simulink model "lab3_nonlinear"  (R2025b)
settings: Solver=VariableStepAuto  StartTime=0.0  StopTime=10.0  RelTol=1e-10  AbsTol=1e-10
values from neighbouring files (symbols this model uses):
  A = double(subs(J1, [x;u], [x_bar;u_bar]))    [lab3.m]
  B = double(subs(J2, [x;u], [x_bar;u_bar]))    [lab3.m]
  K = -K_LQR2    [lab3.m]
  Ulim = 5.875    [lab3.m]
  x0 = [0; 0; 2*pi/24; 0]    [lab3.m]

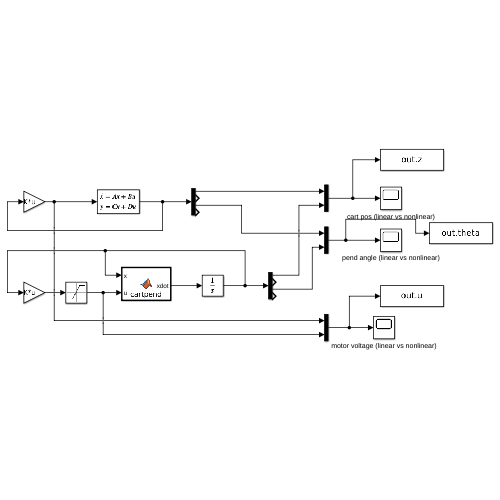
[thumbnail: Simulink's stored preview of the top-level diagram]
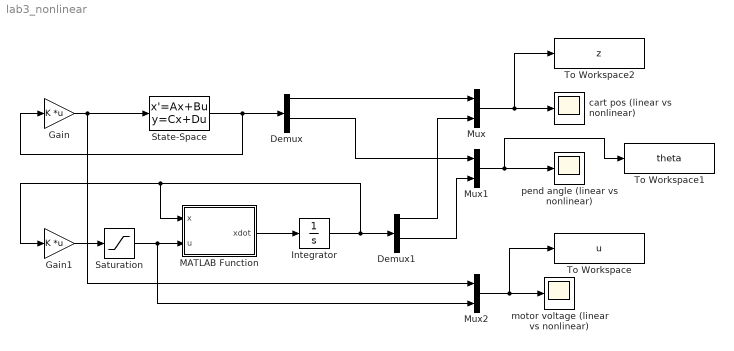
== system lab3_nonlinear ==
  Demux : Demux
  Demux1 : Demux
  Gain : Gain  Gain=K  Multiplication=Matrix(K*u)
  Gain1 : Gain  Gain=K  Multiplication=Matrix(K*u)
  Integrator : Integrator  InitialCondition=x0
  MATLAB Function : MATLAB Function  TreatAsAtomicUnit=on
  Mux : Mux  Inputs=2
  Mux1 : Mux  Inputs=2
  Mux2 : Mux  Inputs=2
  Saturation : Saturate  UpperLimit=Ulim  LowerLimit=-Ulim
  State-Space : StateSpace  A=A  B=B  C=eye(4)  D=zeros(4,1)  InitialCondition=x0
  To Workspace : ToWorkspace  VariableName=u  SaveFormat=Timeseries  SampleTime=-1
  To Workspace1 : ToWorkspace  VariableName=theta  SaveFormat=Timeseries  SampleTime=-1
  To Workspace2 : ToWorkspace  VariableName=z  SaveFormat=Timeseries  SampleTime=-1
  cart pos (linear vs nonlinear) : Scope
      settings: ActiveDisplayYMinimum=-0.12196514215297433  ActiveDisplayYMaximum=-0.023098636726185284
  motor voltage (linear vs nonlinear) : Scope
      settings: DataLoggingVariableName=ScopeData2
  pend angle (linear vs nonlinear) : Scope
      settings: ActiveDisplayYMinimum=-0.089196382902815077  ActiveDisplayYMaximum=0.15535481354428468
  wires:
  Gain/1 -> Mux2/1, State-Space/1
  State-Space/1 -> Gain/1, Demux/1
  Demux/1 -> Mux/1
  Gain1/1 -> Saturation/1
  Saturation/1 -> Mux2/2, MATLAB Function/2(u)
  MATLAB Function/1(xdot) -> Integrator/1
  Integrator/1 -> Demux1/1, Gain1/1, MATLAB Function/1(x)
  Demux/3 -> Mux1/1
  Demux1/1 -> Mux/2
  Demux1/3 -> Mux1/2
  Mux/1 -> To Workspace2/1, cart pos (linear vs nonlinear)/1
  Mux1/1 -> To Workspace1/1, pend angle (linear vs nonlinear)/1
  Mux2/1 -> To Workspace/1, motor voltage (linear vs nonlinear)/1

== matlab function lab3_nonlinear/MATLAB Function ==
  data: x input; u input; xdot output
function xdot = cartpend(x,u)
xdot = cartpend(x,u);
